simulink model "PD_cascade"  (R2021a)
settings: Solver=FixedStepAuto  StartTime=0.0  StopTime=5.0  RelTol=1e-3  EnableMultiTasking=on
undefined symbols (not defined in the file or in its folder): AUX, dev, pwm_output1
libraries: px4Sensorslib x4, cstblocks x3, px4lib x2, simulink x1
settings Model: ExtModeTrigDuration=10  Creator=beket  LastModifiedBy=kawaguchi
settings SolverCC: AlgebraicLoopSolver=TrustRegion  PositivePriorityOrder=on
settings OptimizationCC: EnhancedBackFolding=on  PassReuseOutputArgsAs=Individual arguments  ZeroExternalMemoryAtStartup=off  ZeroInternalMemoryAtStartup=off  MaxStackSize=64  OptimizeBlockOrder=speed  DifferentSizesBufferReuse=on  OptimizationCustomize=off  EfficientTunableParamExpr=on
settings DebuggingCC: ParameterTunabilityLossMsg=error  SymbolicDimsDataTypeCodeGenerationDiagnostic=none  SFMachineParentedDataDiag=warning
settings HardwareCC: ProdBitPerPointer=32  ProdBitPerSizeT=32  ProdBitPerPtrDiffT=32  ProdLargestAtomicInteger=Long  ProdLargestAtomicFloat=Double  ProdWordSize=32  ProdLongLongMode=on  ProdHWDeviceType=ARM Compatible->ARM Cortex
settings SFSimCC: MATLABDynamicMemAlloc=off  SimTargetLang=C++
settings RTWCC: SystemTargetFile=ert.tlc  HardwareBoard=PX4 Pixhawk 4  TLCOptions="-aInlineSetEventsForThisBaseRateFcn=TLC_FALSE -aSuppressMultiTaskScheduler=TLC_FALSE  -aRateBasedStepFcn=0"  TemplateMakefile=ert_default_tmf  Toolchain=GNU Tools for PX4 Autopilots  IncludeHyperlinkInReport=on  TargetLang=C++
settings CodeAppCC: ForceParamTrailComments=on  IgnoreCustomStorageClasses=off  OperatorAnnotations=on  SimulinkDataObjDesc=on  SFDataObjDesc=on  InsertBlockDesc=on
settings ERTTargetCC: ExtModeTransport=3  ExtModeStaticAlloc=on  ExtModeStaticAllocSize=1024  ExtModeMexFile=ext_xcp  ExtModeIntrfLevel=Level2 - Open

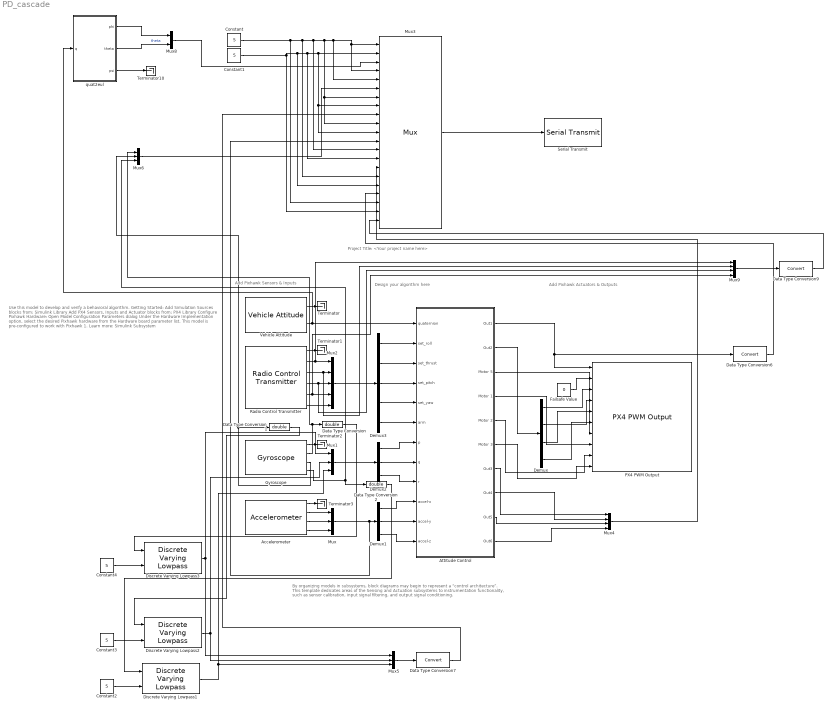
== system PD_cascade ==
  note: Project Title: <Your project name here>
  note: Use this model to develop and verify a behavioral algorithm.
      |
      | Getting Started:
      |
      | Add Simulation Sources blocks from:
      | Simulink Library
      |
      | Add PX4 Sensors, Inputs and Actuator blocks from:
      | PX4 Library
      |
      | Configure Pixhawk Hardware:
      |
      | Open Model Configuration Parameters dialog
      |
      | Under the Hardware Implementation option, select the desired Pixhawk hardware from the Hardware board parameter list.
      |
      | This model is pre-configured to work with Pixhawk 1.
      |
      | Learn more:
      |
      | Simulink Subsystem
  note: Add Pixhawk Sensors & Inputs
  note: Design your algorithm here
  note: Add Pixhawk Actuators & Outputs
  note: By organizing models in subsystems, block diagrams may begin to represent a “control architecture”.
      | This template dedicates areas of the Sensing and Actuation subsystems to instrumentation functionality, such as sensor calibration, input signal filtering, and output signal conditioning.
  Accelerometer : px4Sensorslib/Accelerometer  uorbTimeStamp=off  BlockingMode=off  BlockTimeout=1e-3  sampleTime=1/250
      settings: SourceProductBaseCode=PX4AUTOPILOTS
  Attitude Control : Subsystem
  Constant : Constant  Value=5  OutDataTypeStr=single
  Constant1 : Constant  Value=5  OutDataTypeStr=single
  Constant2 : Constant  Value=5
  Constant3 : Constant  Value=5
  Constant4 : Constant  Value=5
  Data Type Conversion : DataTypeConversion  OutDataTypeStr=double
  Data Type Conversion1 : DataTypeConversion  OutDataTypeStr=double
  Data Type Conversion2 : DataTypeConversion  OutDataTypeStr=double
  Data Type Conversion6 : DataTypeConversion
  Data Type Conversion7 : DataTypeConversion
  Data Type Conversion9 : DataTypeConversion
  Demux : Demux
  Demux1 : Demux  Outputs=3
  Demux2 : Demux  Outputs=3
  Demux3 : Demux  Outputs=5
  Discrete Varying Lowpass1 : cstblocks/Linear Parameter Varying/Discrete Varying Lowpass  N=1  w0=0  Ts=1/250
      settings: SourceProductBaseCode=CT
  Discrete Varying Lowpass2 : cstblocks/Linear Parameter Varying/Discrete Varying Lowpass  N=1  w0=0  Ts=1/250
      settings: SourceProductBaseCode=CT
  Discrete Varying Lowpass3 : cstblocks/Linear Parameter Varying/Discrete Varying Lowpass  N=1  w0=0  Ts=1/250
      settings: SourceProductBaseCode=CT
  Failsafe Value : Constant  Value=0  OutDataTypeStr=boolean  SampleTime=-1
  Gyroscope : px4Sensorslib/Gyroscope  uorbTimeStamp=off  BlockingMode=off  BlockTimeout=1e-3  sampleTime=1/250
      settings: SourceProductBaseCode=PX4AUTOPILOTS
  Mux{,1,5..6} (4 alike) : Mux  Inputs=3
  Mux2 : Mux  Inputs=5
  Mux3 : Mux  Inputs=21
  Mux4 : Mux
  Mux8 : Mux  Inputs=2
  Mux9 : Mux
  PX4 PWM Output : px4lib/PX4 PWM Output  pwmDevice=AUX (/dev/pwm_output1)  pwmChannel1_=on  pwmChannel2_=on  pwmChannel3_=on  pwmChannel4_=on  pwmChannel5_=on  pwmChannel6_=on  pwmChannel7_=on  pwmChannel8_=on  forceTerminateFailsafe=off  outputErrorStatus=off
      settings: SourceProductBaseCode=PX4AUTOPILOTS
  Radio Control Transmitter : px4Sensorslib/Radio Control Transmitter  channel1=on  channel2=on  channel3=on  channel4=on  channel5=on  channel6=off  channel7=off  channel8=off  channel_count=off  rssi=off  rc_input_source=off  timestamp_last_signal=off  time_stamp=off  sampleTime=1/250  BlockingMode=off  BlockTimeout=5
      settings: SourceProductBaseCode=PX4AUTOPILOTS
  Serial Transmit : px4lib/Serial Transmit  SCIModule=/dev/ttyS2
      settings: SourceProductBaseCode=PX4AUTOPILOTS
  Terminator{,1..3,10} (5 alike) : Terminator
  Vehicle Attitude : px4Sensorslib/Vehicle Attitude  rollRate=off  pitchRate=off  yawRate=off  quaternion=on  uorbTimeStamp=off  BlockingMode=off  BlockTimeout=0.001  sampleTime=1/250
      settings: SourceProductBaseCode=PX4AUTOPILOTS
  quat2eul : MATLAB Function  TreatAsAtomicUnit=on
  wires:
  Vehicle Attitude/1 -> Terminator/1
  Radio Control Transmitter/1 -> Terminator1/1
  Gyroscope/1 -> Terminator2/1
  Accelerometer/1 -> Terminator3/1
  Failsafe Value/1 -> PX4 PWM Output/2
  Attitude Control/1(Out1) -> Data Type Conversion6/1, PX4 PWM Output/1
  Attitude Control/2(Out2) -> Demux/1
  Demux/4 -> PX4 PWM Output/6
  Demux/3 -> PX4 PWM Output/5
  Demux/2 -> PX4 PWM Output/4
  Demux/1 -> PX4 PWM Output/3
  Accelerometer/3 -> Mux/2
  Accelerometer/2 -> Mux/1
  Accelerometer/4 -> Mux/3
  Mux/1 -> Mux3/12, Demux1/1
  Demux1/3 -> Attitude Control/12(accel-z)
  Demux1/2 -> Attitude Control/11(accel-y)
  Demux1/1 -> Attitude Control/10(accel-x)
  Mux1/1 -> Demux2/1
  Gyroscope/2 -> Mux6/1, Data Type Conversion/1
  Gyroscope/4 -> Mux6/3, Data Type Conversion2/1
  Demux2/1 -> Attitude Control/7(p)
  Demux2/2 -> Attitude Control/8(q)
  Demux2/3 -> Attitude Control/9(r)
  Mux2/1 -> Demux3/1
  Radio Control Transmitter/2 -> Mux9/1, Mux2/1
  Radio Control Transmitter/3 -> Mux9/2, Mux2/2
  Radio Control Transmitter/4 -> Mux9/3, Mux2/3
  Radio Control Transmitter/5 -> Mux9/4, Mux2/4
  Radio Control Transmitter/6 -> Mux2/5
  Demux3/2 -> Attitude Control/3(set_thrust)
  Demux3/3 -> Attitude Control/4(set_pitch)
  Demux3/1 -> Attitude Control/2(set_roll)
  Demux3/4 -> Attitude Control/5(set_yaw)
  Demux3/5 -> Attitude Control/6(arm)
  Data Type Conversion2/1 -> Discrete Varying Lowpass1/1
  Attitude Control/3(Motor 5) -> PX4 PWM Output/7
  Attitude Control/4(Motor 1) -> PX4 PWM Output/8
  Attitude Control/5(Motor 2) -> PX4 PWM Output/9
  Attitude Control/6(Motor 3) -> PX4 PWM Output/10
  Mux3/1 -> Serial Transmit/1
  Constant/1 -> Mux3/19, Mux3/16, Mux3/13, Mux3/10, Mux3/7, Mux3/5, Mux3/4, Mux3/1
  Constant1/1 -> Mux3/20, Mux3/17, Mux3/14, Mux3/11, Mux3/8, Mux3/2
  Constant2/1 -> Discrete Varying Lowpass1/2
  Discrete Varying Lowpass1/1 -> Mux5/3, Mux1/3
  Data Type Conversion1/1 -> Discrete Varying Lowpass2/1
  Constant3/1 -> Discrete Varying Lowpass2/2
  Discrete Varying Lowpass2/1 -> Mux5/2, Mux1/2
  Data Type Conversion/1 -> Discrete Varying Lowpass3/1
  Constant4/1 -> Discrete Varying Lowpass3/2
  Discrete Varying Lowpass3/1 -> Mux5/1, Mux1/1
  Attitude Control/7(Out3) -> Mux4/1
  Attitude Control/8(Out4) -> Mux4/2
  Attitude Control/9(Out5) -> Mux4/3
  Attitude Control/10(Out6) -> Mux4/4
  Gyroscope/3 -> Mux6/2, Data Type Conversion1/1
  Mux6/1 -> Mux3/6
  Data Type Conversion9/1 -> Mux3/21
  Data Type Conversion6/1 -> Mux3/18
  Mux4/1 -> Mux3/15
  Mux8/1 -> Mux3/3
  quat2eul/3(psi) -> Terminator10/1
  quat2eul/2(theta) -> Mux8/2  "theta"
  Vehicle Attitude/2 -> quat2eul/1(q), Attitude Control/1(quaternion)
  quat2eul/1(phi) -> Mux8/1
  Mux5/1 -> Data Type Conversion7/1
  Data Type Conversion7/1 -> Mux3/9
  Mux9/1 -> Data Type Conversion9/1

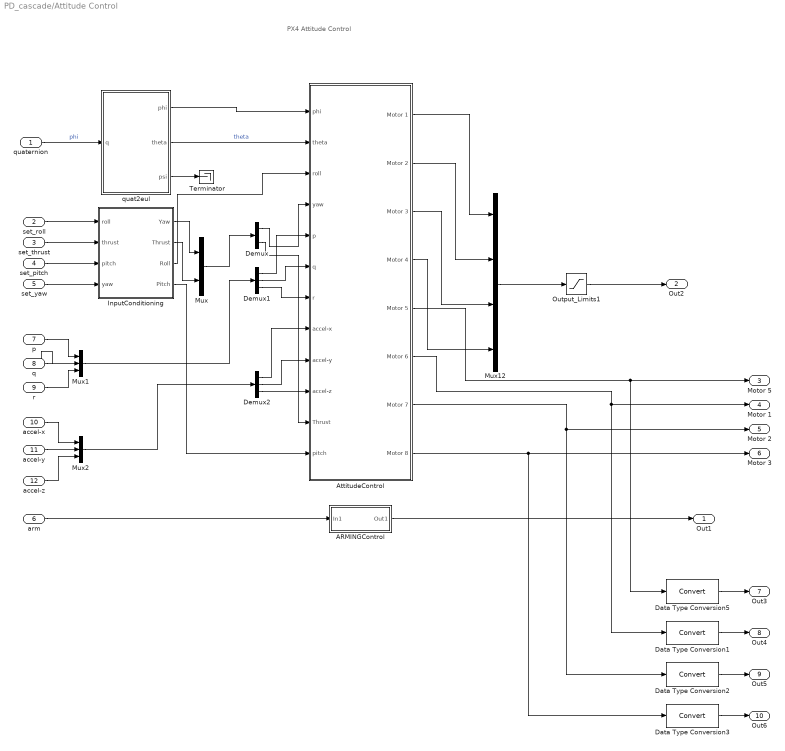
== system PD_cascade/Attitude Control ==
  note: PX4 Attitude Control
  quaternion : Inport
  set_roll : Inport  Port=2  OutDataTypeStr=uint16
  set_thrust : Inport  Port=3  OutDataTypeStr=uint16
  set_pitch : Inport  Port=4  OutDataTypeStr=uint16
  set_yaw : Inport  Port=5  OutDataTypeStr=uint16
  arm : Inport  Port=6  OutDataTypeStr=uint16
  p : Inport  Port=7
  q : Inport  Port=8
  r : Inport  Port=9
  accel-x : Inport  Port=10
  accel-y : Inport  Port=11
  accel-z : Inport  Port=12
  ARMINGControl : Subsystem
  AttitudeControl : Subsystem
  Data Type Conversion{1..3,5} (4 alike) : DataTypeConversion
  Demux : Demux  Outputs=2
  Demux1 : Demux  Outputs=3
  Demux2 : Demux  Outputs=3
  InputConditioning : Subsystem
  Mux : Mux  Inputs=2
  Mux1 : Mux  Inputs=3
  Mux12 : Mux
  Mux2 : Mux  Inputs=3
  Output_Limits1 : Saturate  UpperLimit=2000  LowerLimit=1000
  Terminator : Terminator
  quat2eul : MATLAB Function  TreatAsAtomicUnit=on
  Out1 : Outport  VectorParamsAs1DForOutWhenUnconnected=off
  Out2 : Outport  Port=2  VectorParamsAs1DForOutWhenUnconnected=off
  Motor 5 : Outport  Port=3  OutDataTypeStr=uint16  VectorParamsAs1DForOutWhenUnconnected=off
  Motor 1 : Outport  Port=4  OutDataTypeStr=uint16  VectorParamsAs1DForOutWhenUnconnected=off
  Motor 2 : Outport  Port=5  OutDataTypeStr=uint16  VectorParamsAs1DForOutWhenUnconnected=off
  Motor 3 : Outport  Port=6  OutDataTypeStr=uint16  VectorParamsAs1DForOutWhenUnconnected=off
  Out3 : Outport  Port=7
  Out4 : Outport  Port=8
  Out5 : Outport  Port=9
  Out6 : Outport  Port=10
  wires:
  set_roll/1 -> InputConditioning/1(roll)
  arm/1 -> ARMINGControl/1(In1)
  quat2eul/2(theta) -> AttitudeControl/2(theta)  "theta"
  Output_Limits1/1 -> Out2/1
  Mux12/1 -> Output_Limits1/1
  ARMINGControl/1(Out1) -> Out1/1
  set_yaw/1 -> InputConditioning/4(yaw)
  quaternion/1 -> quat2eul/1(q)  "phi"
  quat2eul/1(phi) -> AttitudeControl/1(phi)
  quat2eul/3(psi) -> Terminator/1
  AttitudeControl/1(Motor 1) -> Mux12/1
  AttitudeControl/2(Motor 2) -> Mux12/2
  AttitudeControl/3(Motor 3) -> Mux12/3
  AttitudeControl/4(Motor 4) -> Mux12/4
  Mux/1 -> Demux/1
  p/1 -> Mux1/1
  r/1 -> Mux1/3
  Mux1/1 -> Demux1/1
  Demux1/2 -> AttitudeControl/6(q)
  Demux1/1 -> AttitudeControl/5(p)
  Demux1/3 -> AttitudeControl/7(r)
  accel-y/1 -> Mux2/2
  accel-x/1 -> Mux2/1
  accel-z/1 -> Mux2/3
  Mux2/1 -> Demux2/1
  Demux2/2 -> AttitudeControl/9(accel-y)
  Demux2/1 -> AttitudeControl/8(accel-x)
  Demux2/3 -> AttitudeControl/10(accel-z)
  InputConditioning/1(Yaw) -> Mux/1
  InputConditioning/2(Thrust) -> Mux/2
  Demux/1 -> AttitudeControl/4(yaw)
  Demux/2 -> AttitudeControl/11(Thrust)
  InputConditioning/3(Roll) -> AttitudeControl/3(roll)
  InputConditioning/4(Pitch) -> AttitudeControl/12(pitch)
  AttitudeControl/5(Motor 5) -> Data Type Conversion5/1, Motor 5/1
  set_thrust/1 -> InputConditioning/2(thrust)
  set_pitch/1 -> InputConditioning/3(pitch)
  AttitudeControl/6(Motor 6) -> Data Type Conversion1/1, Motor 1/1
  AttitudeControl/7(Motor 7) -> Data Type Conversion2/1, Motor 2/1
  AttitudeControl/8(Motor 8) -> Data Type Conversion3/1, Motor 3/1
  q/1 -> Mux1/2
  Data Type Conversion5/1 -> Out3/1
  Data Type Conversion1/1 -> Out4/1
  Data Type Conversion2/1 -> Out5/1
  Data Type Conversion3/1 -> Out6/1

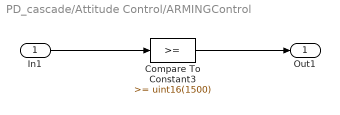
== system PD_cascade/Attitude Control/ARMINGControl ==
  In1 : Inport
  Compare To Constant3 : simulink/Logic and Bit Operations/Compare To Constant  relop=>=  const=uint16(1500)  OutDataTypeStr=boolean
  Out1 : Outport  VectorParamsAs1DForOutWhenUnconnected=off
  wires:
  Compare To Constant3/1 -> Out1/1
  In1/1 -> Compare To Constant3/1

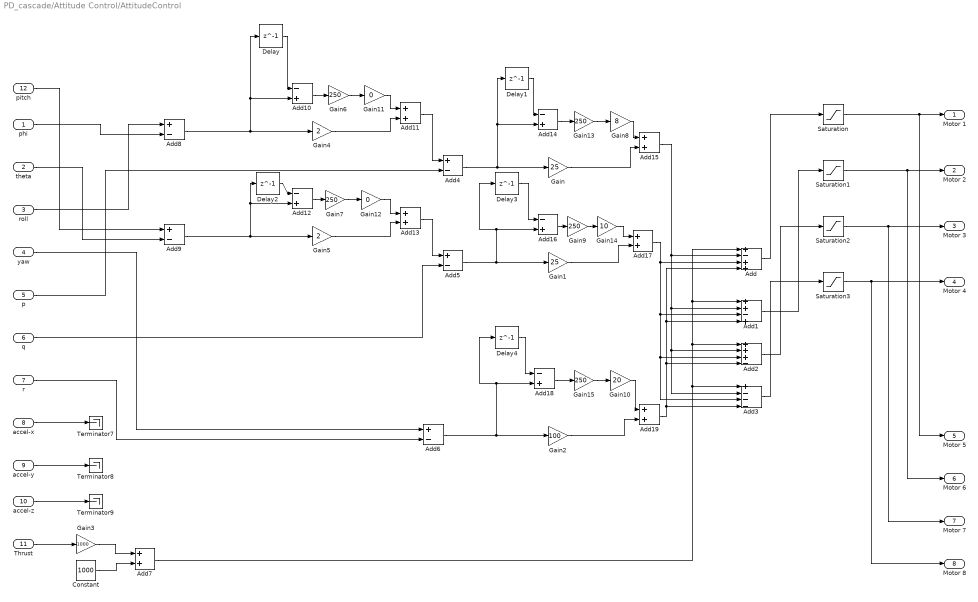
== system PD_cascade/Attitude Control/AttitudeControl ==
  phi : Inport
  theta : Inport  Port=2
  roll : Inport  Port=3
  yaw : Inport  Port=4
  p : Inport  Port=5
  q : Inport  Port=6
  r : Inport  Port=7
  accel-x : Inport  Port=8
  accel-y : Inport  Port=9
  accel-z : Inport  Port=10
  Thrust : Inport  Port=11
  pitch : Inport  Port=12
  Add : Sum  Inputs=+-++
  Add1 : Sum  Inputs=++-+
  Add{10,12,14,16,18} (5 alike) : Sum  Inputs=-+
  Add{7,11,13,15,17,19} (6 alike) : Sum
  Add2 : Sum  Inputs=+++-
  Add3 : Sum  Inputs=+---
  Add{4..6,8..9} (5 alike) : Sum  Inputs=+-
  Constant : Constant  Value=1000
  Delay{,1..4} (5 alike) : Delay  DelayLength=1  InitialCondition=0
  Gain : Gain  Gain=25
  Gain1 : Gain  Gain=25
  Gain10 : Gain  Gain=20
  Gain11 : Gain  Gain=0
  Gain12 : Gain  Gain=0
  Gain{6..7,9,13,15} (5 alike) : Gain  Gain=250
  Gain14 : Gain  Gain=10
  Gain2 : Gain  Gain=100
  Gain3 : Gain  Gain=1000
  Gain4 : Gain  Gain=2
  Gain5 : Gain  Gain=2
  Gain8 : Gain  Gain=8
  Saturation{,1..3} (4 alike) : Saturate  UpperLimit=2000  LowerLimit=800  OutDataTypeStr=uint16
  Terminator7 : Terminator
  Terminator8 : Terminator
  Terminator9 : Terminator
  Motor 1 : Outport  OutDataTypeStr=uint16  VectorParamsAs1DForOutWhenUnconnected=off
  Motor 2 : Outport  Port=2  OutDataTypeStr=uint16  VectorParamsAs1DForOutWhenUnconnected=off
  Motor 3 : Outport  Port=3  OutDataTypeStr=uint16  VectorParamsAs1DForOutWhenUnconnected=off
  Motor 4 : Outport  Port=4  OutDataTypeStr=uint16  VectorParamsAs1DForOutWhenUnconnected=off
  Motor 5 : Outport  Port=5  OutDataTypeStr=uint16  SampleTime=1/250  VectorParamsAs1DForOutWhenUnconnected=off
  Motor 6 : Outport  Port=6  OutDataTypeStr=uint16  VectorParamsAs1DForOutWhenUnconnected=off
  Motor 7 : Outport  Port=7  OutDataTypeStr=uint16  VectorParamsAs1DForOutWhenUnconnected=off
  Motor 8 : Outport  Port=8  OutDataTypeStr=uint16  VectorParamsAs1DForOutWhenUnconnected=off
  wires:
  Add2/1 -> Saturation2/1
  Gain/1 -> Add15/2
  Add17/1 -> Add2/3, Add3/3, Add1/3, Add/3
  Add18/1 -> Gain15/1
  Add13/1 -> Add5/1
  Add14/1 -> Gain13/1
  Gain15/1 -> Gain10/1
  Gain11/1 -> Add11/1
  Gain1/1 -> Add17/2
  Gain3/1 -> Add7/1
  theta/1 -> Add9/2
  Gain14/1 -> Add17/1
  Gain12/1 -> Add13/1
  Gain5/1 -> Add13/2
  Saturation/1 -> Motor 5/1, Motor 1/1
  r/1 -> Add6/2
  Gain9/1 -> Gain14/1
  Gain13/1 -> Gain8/1
  Gain7/1 -> Gain12/1
  Add19/1 -> Add3/4, Add2/4, Add1/4, Add/4
  Add15/1 -> Add/2, Add1/2, Add2/2, Add3/2
  Add16/1 -> Gain9/1
  accel-z/1 -> Terminator9/1
  Delay3/1 -> Add16/1
  Constant/1 -> Add7/2
  Gain10/1 -> Add19/1
  Delay/1 -> Add10/1
  Gain4/1 -> Add11/2
  Add5/1 -> Delay3/1, Add16/2, Gain1/1
  Gain6/1 -> Gain11/1
  Thrust/1 -> Gain3/1
  Delay4/1 -> Add18/1
  Add8/1 -> Gain4/1, Delay/1, Add10/2
  Delay2/1 -> Add12/1
  Add11/1 -> Add4/1
  Add12/1 -> Gain7/1
  accel-x/1 -> Terminator7/1
  Add4/1 -> Gain/1, Delay1/1, Add14/2
  Add3/1 -> Saturation3/1
  Gain2/1 -> Add19/2
  Saturation2/1 -> Motor 7/1, Motor 3/1
  Add6/1 -> Delay4/1, Add18/2, Gain2/1
  Add/1 -> Saturation/1
  Add10/1 -> Gain6/1
  roll/1 -> Add8/1
  phi/1 -> Add8/2
  pitch/1 -> Add9/1
  Saturation3/1 -> Motor 8/1, Motor 4/1
  Add9/1 -> Delay2/1, Add12/2, Gain5/1
  Add1/1 -> Saturation1/1
  Add7/1 -> Add/1, Add1/1, Add2/1, Add3/1
  accel-y/1 -> Terminator8/1
  Saturation1/1 -> Motor 6/1, Motor 2/1
  p/1 -> Add4/2
  q/1 -> Add5/2
  Gain8/1 -> Add15/1
  yaw/1 -> Add6/1
  Delay1/1 -> Add14/1

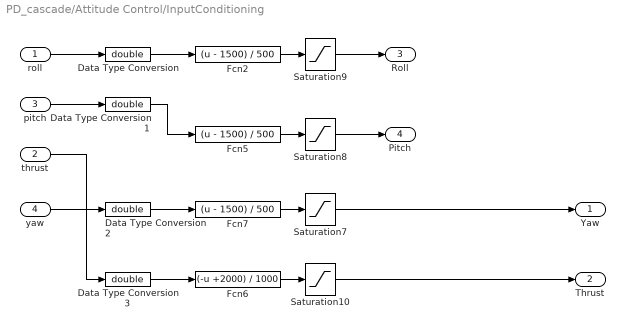
== system PD_cascade/Attitude Control/InputConditioning ==
  roll : Inport
  thrust : Inport  Port=2
  pitch : Inport  Port=3
  yaw : Inport  Port=4
  Data Type Conversion{,1..3} (4 alike) : DataTypeConversion  OutDataTypeStr=double
  Fcn2 : Fcn  Expr=(u - 1500) / 500
  Fcn5 : Fcn  Expr=(u - 1500) / 500
  Fcn6 : Fcn  Expr=(-u +2000) / 1000
  Fcn7 : Fcn  Expr=(u - 1500) / 500
  Saturation10 : Saturate  UpperLimit=1  LowerLimit=0
  Saturation7 : Saturate  UpperLimit=1  LowerLimit=-1
  Saturation8 : Saturate  UpperLimit=1  LowerLimit=-1
  Saturation9 : Saturate  UpperLimit=1  LowerLimit=-1
  Yaw : Outport  VectorParamsAs1DForOutWhenUnconnected=off
  Thrust : Outport  Port=2  VectorParamsAs1DForOutWhenUnconnected=off
  Roll : Outport  Port=3  VectorParamsAs1DForOutWhenUnconnected=off
  Pitch : Outport  Port=4  VectorParamsAs1DForOutWhenUnconnected=off
  wires:
  Saturation10/1 -> Thrust/1
  Saturation7/1 -> Yaw/1
  Saturation8/1 -> Pitch/1
  Fcn6/1 -> Saturation10/1
  thrust/1 -> Data Type Conversion3/1
  Fcn2/1 -> Saturation9/1
  Fcn5/1 -> Saturation8/1
  Saturation9/1 -> Roll/1
  Fcn7/1 -> Saturation7/1
  yaw/1 -> Data Type Conversion2/1
  pitch/1 -> Data Type Conversion1/1
  roll/1 -> Data Type Conversion/1
  Data Type Conversion/1 -> Fcn2/1
  Data Type Conversion1/1 -> Fcn5/1
  Data Type Conversion2/1 -> Fcn7/1
  Data Type Conversion3/1 -> Fcn6/1

== matlab function PD_cascade/Attitude Control/quat2eul ==
  data: q input; phi output; theta output; psi output
function [phi,theta,psi] = quat2eul(q)

% Quaternion conversion to Euler angles based on the PX4 Firmware v1.6.5
% release.

phi = atan2(2*(q(1)*q(2) + q(3)* q(4)), q(1)^2 - q(2)^2 - q(3)^2 + q(4)^2);
theta = asin(-2*(q(2)*q(4) - q(1)*q(3)));
psi = atan2(2*(q(2)*q(3) + q(1)* q(4)), q(1)^2 + q(2)^2 - q(3)^2 - q(4)^2);

end

== matlab function PD_cascade/quat2eul ==
  data: q input; phi output; theta output; psi output
function [phi,theta,psi] = quat2eul(q)

% Quaternion conversion to Euler angles based on the PX4 Firmware v1.6.5
% release.

phi = atan2(2*(q(1)*q(2) + q(3)* q(4)), q(1)^2 - q(2)^2 - q(3)^2 + q(4)^2);
theta = asin(-2*(q(2)*q(4) - q(1)*q(3)));
psi = atan2(2*(q(2)*q(3) + q(1)* q(4)), q(1)^2 + q(2)^2 - q(3)^2 - q(4)^2);

end
